simulink model "base"  (R2017b)
settings: Solver=VariableStepAuto  StartTime=0.0  StopTime=1600  RelTol=1e-3
InitFcn:
  | A=[0 1;5 -6];
  | b=[4;4];
  | C=[2 3];
  | U=ctrb(A,b);
  | rank(U);
  | Ad=[0 1;-256 -32];
  | H=[1 0];
  | U2=obsv(Ad,H);
  | rank(U2);
  | 
  | M=sylv(A,-Ad,b*H);
  | K=H*inv(M);
  | 
  | k0g=0.02;
  | k1g=1;
  | k2g=3;
  | k3g=5;
  | A0g=[0 1 0 0;
  |      0 0 1 0;
  |      0 0 0 1;
  |      -k0g -k1g -k2g -k3g ];
  | b0g=[0;0;0;1];
  | 
  | Am=A-b*K;
settings Model: Creator=lida  LastModifiedBy=lida

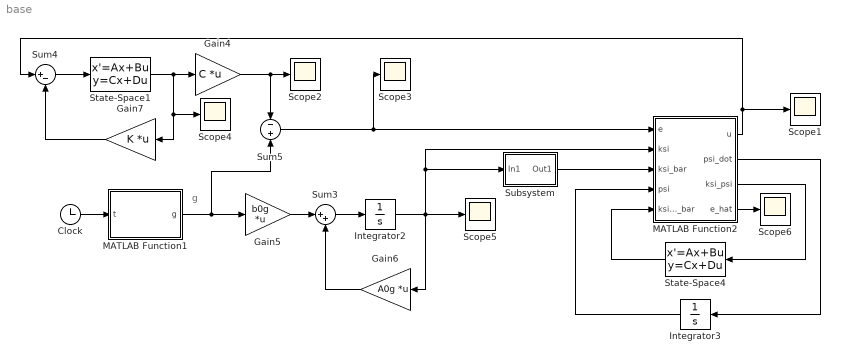
== system base ==
  note: g
  Clock : Clock
  Gain4 : Gain  Gain=C  Multiplication=Matrix(K*u)
  Gain5 : Gain  Gain=b0g  Multiplication=Matrix(K*u)
  Gain6 : Gain  Gain=A0g  Multiplication=Matrix(K*u)
  Gain7 : Gain  Gain=K  Multiplication=Matrix(K*u)
  Integrator2 : Integrator  InitialCondition=[0;0;0;0]
  Integrator3 : Integrator  InitialCondition=[0;0;0;0]
  MATLAB Function1 : MATLAB Function  TreatAsAtomicUnit=on
  MATLAB Function2 : MATLAB Function  TreatAsAtomicUnit=on
  Scope{1..6} (6 alike) : Scope
  State-Space1 : StateSpace  A=A  B=b  C=eye(2)  D=[0;0]  InitialCondition=[1;0]
  State-Space4 : StateSpace  A=Am  B=b  C=C  D=0  InitialCondition=0
  Subsystem : Subsystem
  Sum3 : Sum  Inputs=|++
  Sum4 : Sum  Inputs=|+-
  Sum5 : Sum  Inputs=-+
  wires:
  Clock/1 -> MATLAB Function1/1(t)
  State-Space1/1 -> Gain7/1, Scope4/1, Gain4/1
  MATLAB Function1/1(g) -> Sum5/2, Gain5/1
  Gain5/1 -> Sum3/1
  Sum3/1 -> Integrator2/1
  Integrator2/1 -> Scope5/1, Subsystem/1(In1), MATLAB Function2/2(ksi), Gain6/1
  Gain6/1 -> Sum3/2
  Sum4/1 -> State-Space1/1
  Gain7/1 -> Sum4/2
  Gain4/1 -> Sum5/1, Scope2/1
  Sum5/1 -> Scope3/1, MATLAB Function2/1(e)
  Subsystem/1(Out1) -> MATLAB Function2/3(ksi_bar)
  MATLAB Function2/3(ksi_psi) -> State-Space4/1
  State-Space4/1 -> MATLAB Function2/5(ksi_psi_bar)
  MATLAB Function2/2(psi_dot) -> Integrator3/1
  Integrator3/1 -> MATLAB Function2/4(psi)
  MATLAB Function2/1(u) -> Sum4/1, Scope1/1
  MATLAB Function2/4(e_hat) -> Scope6/1

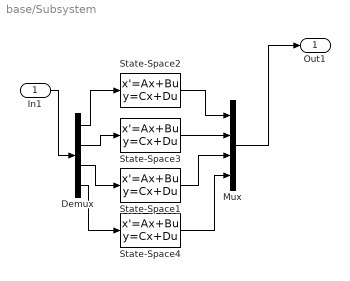
== system base/Subsystem ==
  In1 : Inport
  Demux : Demux
  Mux : Mux
  State-Space{1..4} (4 alike) : StateSpace  A=Am  B=b  C=C  D=0  InitialCondition=0
  Out1 : Outport
  wires:
  In1/1 -> Demux/1
  Demux/1 -> State-Space2/1
  Mux/1 -> Out1/1
  State-Space2/1 -> Mux/1
  State-Space3/1 -> Mux/2
  Demux/2 -> State-Space3/1
  Demux/3 -> State-Space1/1
  Demux/4 -> State-Space4/1
  State-Space1/1 -> Mux/3
  State-Space4/1 -> Mux/4

== matlab function base/MATLAB Function1 ==
  data: t input; g output
function g = fcn(t)

g=5*sin(3*t-2)*sin(6*t+10);

== matlab function base/MATLAB Function2 ==
  data: e input; u output; ksi input; ksi_bar input; psi_dot output; ksi_psi output; psi input; ksi_psi_bar input; e_hat output
function [u,psi_dot,ksi_psi,e_hat] = fcn(e,ksi,ksi_bar,psi, ksi_psi_bar)
gamma=10000;

e_hat=e-psi'*ksi_bar+ksi_psi_bar;
ksi_psi=ksi'*psi;

psi_dot=gamma*ksi_bar*e_hat;

u=psi'*ksi;
